simulink subsystem "Plant_Model_LTHT_Cooling"  (R2023a)
settings: Solver=VariableStepAuto  StartTime=0.0  StopTime=10.0  RelTol=1e-3
values from neighbouring files (symbols this model uses):
  air_cp = 1004    [All_Properties.mat]    (also in cathode_subsystem_parameters.m; thermal_subsystem_parameters.m)
  air_HC_min = 10    [All_Properties.mat]    (also in cathode_subsystem_parameters.m; thermal_subsystem_parameters.m)
  air_HC_nom = 100    [All_Properties.mat]    (also in cathode_subsystem_parameters.m; thermal_subsystem_parameters.m)
  air_rho = 1.2    [All_Properties.mat]    (also in cathode_subsystem_parameters.m; thermal_subsystem_parameters.m)
  air_vel_nom = 1    [All_Properties.mat]    (also in cathode_subsystem_parameters.m; thermal_subsystem_parameters.m)
  coolant_initial_pressure = 0.111325    [All_Properties.mat]    (also in cathode_subsystem_parameters.m; thermal_subsystem_parameters.m)
  coolant_initial_temperature = 313.15    [All_Properties.mat]    (also in cathode_subsystem_parameters.m = 293.15; thermal_subsystem_parameters.m = 293.15)
  coolant_tube_D = 0.05    [All_Properties.mat]    (also in Plant_Model_HT_Cooling_Parameters.m; cathode_subsystem_parameters.m; environment_parameters.m; stack_model_harness_parameters.m)
  radiator_area_air = 0.1026    [All_Properties.mat]    (also in cathode_subsystem_parameters.m; thermal_subsystem_parameters.m)
  radiator_area_fins = 2.543625    [All_Properties.mat]    (also in cathode_subsystem_parameters.m; thermal_subsystem_parameters.m)
  radiator_area_primary = 0.444525    [All_Properties.mat]    (also in cathode_subsystem_parameters.m; thermal_subsystem_parameters.m = 2 * radiator_tube_length * radiator_width * (radiator_fin_ro)
  radiator_n_tubes = 20    [All_Properties.mat]    (also in cathode_subsystem_parameters.m; thermal_subsystem_parameters.m)
  radiator_tube_height = 0.0015    [All_Properties.mat]    (also in cathode_subsystem_parameters.m; thermal_subsystem_parameters.m)
  radiator_tube_length = 0.45    [All_Properties.mat]    (also in cathode_subsystem_parameters.m; thermal_subsystem_parameters.m)
  radiator_width = 0.025    [All_Properties.mat]    (also in cathode_subsystem_parameters.m; thermal_subsystem_parameters.m)
  tcp_time_constant = 2    [All_Properties.mat]    (also in Plant_Model_HT_Cooling_Parameters.m; cathode_subsystem_parameters.m; thermal_subsystem_parameters.m)
  tcv_orifice_diameter = 0.045    [All_Properties.mat]    (also in Plant_Model_HT_Cooling_Parameters.m; cathode_subsystem_parameters.m; thermal_subsystem_parameters.m)
  tcv_time_constant = 0.2    [All_Properties.mat]    (also in Plant_Model_HT_Cooling_Parameters.m; cathode_subsystem_parameters.m; thermal_subsystem_parameters.m)
libraries: fl_lib x78, nesl_utility x61, SimscapeFluids_lib x9
(part 2 of 2)

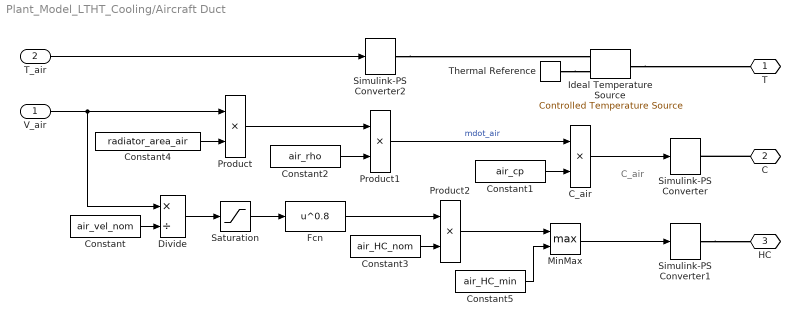
== system Plant_Model_LTHT_Cooling/Aircraft Duct ==
  note: C_air
  V_air : Inport
  T_air : Inport  Port=2
  C_air : Product
  Constant : Constant  Value=air_vel_nom
  Constant1 : Constant  Value=air_cp
  Constant2 : Constant  Value=air_rho
  Constant3 : Constant  Value=air_HC_nom
  Constant4 : Constant  Value=radiator_area_air
  Constant5 : Constant  Value=air_HC_min
  Divide : Product  Inputs=*/
  Fcn : Fcn  Expr=u^0.8
  Ideal Temperature Source : fl_lib/Thermal/Thermal Sources/Controlled Temperature Source
  MinMax : MinMax  Function=max  Inputs=2
  Product : Product
  Product1 : Product
  Product2 : Product
  Saturation : Saturate  UpperLimit=inf  LowerLimit=0
  Simulink-PS Converter : nesl_utility/Simulink-PS Converter  PhysicalDomain=network_engine_domain  SubClassName=ps_input  LeftPortType=input  RightPortType=output  PseudoPeriodic=off  Frequencies=[]  NoiseDistribution=none  NoiseParameters=[]  Unit=W/K  AffineConversion=off  FilteringAndDerivatives=zero  SimscapeFilterOrder=1  InputFilterTimeConstant=1  UdotUserProvided=1
  Simulink-PS Converter1 : nesl_utility/Simulink-PS Converter  PhysicalDomain=network_engine_domain  SubClassName=ps_input  LeftPortType=input  RightPortType=output  PseudoPeriodic=off  Frequencies=[]  NoiseDistribution=none  NoiseParameters=[]  Unit=W/(m^2*K)  AffineConversion=off  FilteringAndDerivatives=zero  SimscapeFilterOrder=1  InputFilterTimeConstant=1  UdotUserProvided=1
  Simulink-PS Converter2 : nesl_utility/Simulink-PS Converter  PhysicalDomain=network_engine_domain  SubClassName=ps_input  LeftPortType=input  RightPortType=output  PseudoPeriodic=off  Frequencies=[]  NoiseDistribution=none  NoiseParameters=[]  Unit=K  AffineConversion=on  FilteringAndDerivatives=zero  SimscapeFilterOrder=1  InputFilterTimeConstant=1  UdotUserProvided=1
  Thermal Reference : fl_lib/Thermal/Thermal Elements/Thermal Reference
  T : PMIOPort  Side=Right
  C : PMIOPort  Port=2  Side=Right
  HC : PMIOPort  Port=3  Side=Right
  wires:
  Saturation/1 -> Fcn/1
  Product1/1 -> C_air/1  "mdot_air"
  Constant4/1 -> Product/2
  Constant2/1 -> Product1/2
  Product/1 -> Product1/1
  C_air/1 -> Simulink-PS Converter/1
  Constant1/1 -> C_air/2
  T_air/1 -> Simulink-PS Converter2/1
  MinMax/1 -> Simulink-PS Converter1/1
  Constant5/1 -> MinMax/2
  Product2/1 -> MinMax/1
  Fcn/1 -> Product2/1
  Divide/1 -> Saturation/1
  Constant3/1 -> Product2/2
  Constant/1 -> Divide/2
  V_air/1 -> Divide/1, Product/1
  connections:
  Ideal Temperature Source/LConn1 -- T/RConn1
  Simulink-PS Converter2/RConn1 -- Ideal Temperature Source/RConn1
  Thermal Reference/LConn1 -- Ideal Temperature Source/RConn2
  Simulink-PS Converter1/RConn1 -- HC/RConn1
  C/RConn1 -- Simulink-PS Converter/RConn1

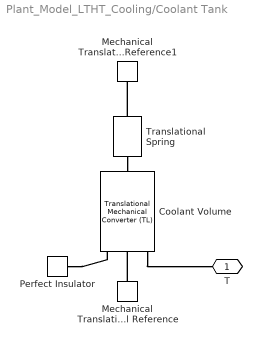
== system Plant_Model_LTHT_Cooling/Coolant Tank ==
  Coolant Volume : fl_lib/Thermal Liquid/Elements/Translational Mechanical Converter (TL)  mech_orientation=foundation.enum.MechOrientationTranslational.Positive  displacement_spec=foundation.enum.DisplacementSpec.Calculate  x0=x_init m  interface_area=A m^2  dead_volume=A * 0.001 m^3  environment_spec=foundation.enum.pressure_spec.specified  environment_pressure=coolant_initial_pressure MPa  dynamic_compressibility=simscape.enum.onoff.off  p0=env_p MPa  T0=coolant_initial_temperature K
      settings: InternalSimscapePortConfiguration="{\"Bottom\":[],\"Left\":[{\"id\":\"A\",\"label\":\"A\",\"type\":\"foundation.thermal_liquid.thermal_liquid\"},{\"id\":\"C\",\"label\":\"C\",\"type\":\"foundation.mechanical.translational.translational\"},{\"id\":\"H\",\"label\":\"H\",\"type\":\"foundation.thermal.thermal\"}],\"Right\":[{\"id\":\"R\",\"label\":\"R\",\"type\":\"foundation.mechanical.translational.translational\"}],\"Top\":[]}"
  Mechanical Translational Reference : fl_lib/Mechanical/Translational Elements/Mechanical Translational Reference
  Mechanical Translational Reference1 : fl_lib/Mechanical/Translational Elements/Mechanical Translational Reference
  Perfect Insulator : fl_lib/Thermal/Thermal Elements/Perfect Insulator  T_specify=off  T_priority=None  T=0 K  T_nominal_specify=off  T_nominal_unit=K  T_nominal_value=1
  Translational Spring : fl_lib/Mechanical/Translational Elements/Translational Spring  spr_rate=1e6 N/m  v_specify=off  v_priority=None  v=0 m/s  v_nominal_specify=off  v_nominal_unit=m/s  v_nominal_value=1  f_specify=off  f_priority=None  f=0 N  f_nominal_specify=off  f_nominal_unit=N  f_nominal_value=1  x_specify=off  x_priority=High  x=x_init m  x_nominal_specify=on  x_nominal_unit=m  x_nominal_value=x_init
  T : PMIOPort  Side=Right
  connections:
  Translational Spring/LConn1 -- Mechanical Translational Reference1/LConn1
  Translational Spring/RConn1 -- Coolant Volume/RConn1
  Perfect Insulator/LConn1 -- Coolant Volume/LConn3
  Mechanical Translational Reference/LConn1 -- Coolant Volume/LConn2
  Coolant Volume/LConn1 -- T/RConn1

== system Plant_Model_LTHT_Cooling/Kelvin to °C ==
  Temp. (K) : Inport
  Constant : Constant  Value=273.15
  Sum : Sum  Inputs=|+-
  Temp. (°C) : Outport
  wires:
  Temp. (K)/1 -> Sum/1
  Sum/1 -> Temp. (°C)/1
  Constant/1 -> Sum/2

== system Plant_Model_LTHT_Cooling/Kelvin to °C1 ==
  Temp. (K) : Inport
  Constant : Constant  Value=273.15
  Sum : Sum  Inputs=|+-
  Temp. (°C) : Outport
  wires:
  Temp. (K)/1 -> Sum/1
  Sum/1 -> Temp. (°C)/1
  Constant/1 -> Sum/2

== system Plant_Model_LTHT_Cooling/Kelvin to °C2 ==
  Temp. (K) : Inport
  Constant : Constant  Value=273.15
  Sum : Sum  Inputs=|+-
  Temp. (°C) : Outport
  wires:
  Temp. (K)/1 -> Sum/1
  Sum/1 -> Temp. (°C)/1
  Constant/1 -> Sum/2

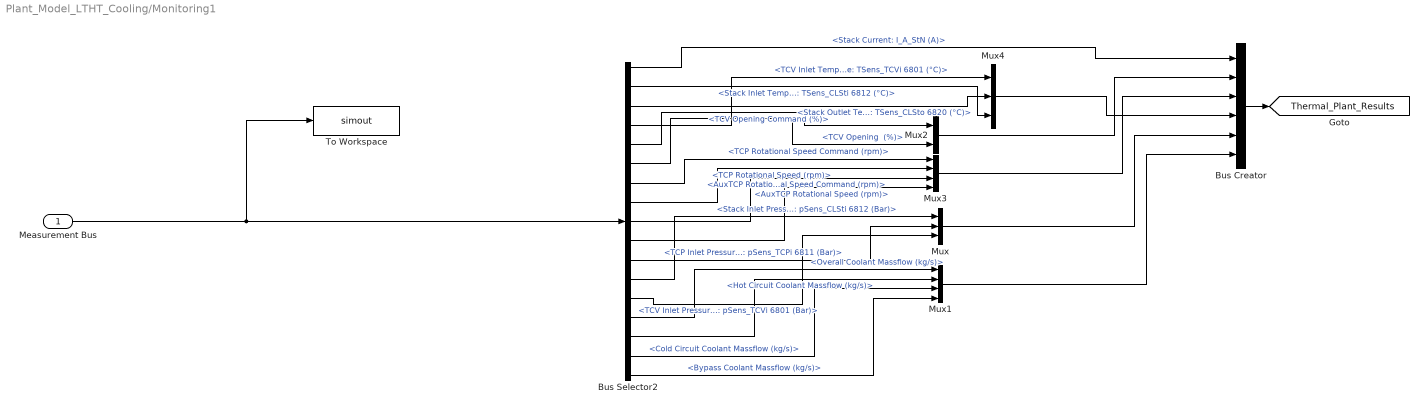
== system Plant_Model_LTHT_Cooling/Monitoring1 ==
  Measurement Bus : Inport
  Bus Creator : BusCreator  Inputs=6
  Bus Selector2 : BusSelector  OutputSignals="Stack Current: I_A_StN (A),Stack Inlet Temperature: TSens_CLSti 6812 (°C),Stack Outlet Temperature: TSens_CLSto 6820 (°C),TCV Inlet Temperature: TSens_TCVi 6801 (°C),TCV Opening Command (%),TCV Opening  (%),TCP Rotational Speed Command (rpm),TCP Rotational Speed (rpm),AuxTCP Rotational Speed Command (rpm),AuxTCP Rotational Speed (rpm),TCP Inlet Pressure: pSens_TCPi 6811 (Bar),Stack Inlet Pressure: pSens_CLSti 6812 (Bar),TCV Inlet Pressure: pSens_TCVi 6801 (Bar),Overall Coolant Massflow (kg/s),Hot Circuit Coolant Massflow (kg/s),Cold Circuit Coolant Massflow (kg/s),Bypass Coolant Massflow (kg/s)"
  Mux : Mux  Inputs=3
  Mux1 : Mux
  Mux2 : Mux  Inputs=2
  Mux3 : Mux
  Mux4 : Mux  Inputs=3
  To Workspace : ToWorkspace  VariableName=simout  SaveFormat=Timeseries  SampleTime=-1
  tag scope: Thermal_Plant_Results=global
  wires:
  Bus Creator/1 -> [Thermal_Plant_Results]
  Bus Selector2/4 -> Mux4/1  "<TCV Inlet Temperature: TSens_TCVi 6801 (°C)>"
  Bus Selector2/1 -> Bus Creator/1  "<Stack Current: I_A_StN (A)>"
  Bus Selector2/12 -> Mux/1  "<Stack Inlet Pressure: pSens_CLSti 6812 (Bar)>"
  Bus Selector2/16 -> Mux1/3  "<Cold Circuit Coolant Massflow (kg/s)>"
  Bus Selector2/5 -> Mux2/1  "<TCV Opening Command (%)>"
  Bus Selector2/8 -> Mux3/2  "<TCP Rotational Speed (rpm)>"
  Bus Selector2/17 -> Mux1/4  "<Bypass Coolant Massflow (kg/s)>"
  Mux1/1 -> Bus Creator/6
  Bus Selector2/14 -> Mux1/1  "<Overall Coolant Massflow (kg/s)>"
  Bus Selector2/13 -> Mux/3  "<TCV Inlet Pressure: pSens_TCVi 6801 (Bar)>"
  Bus Selector2/15 -> Mux1/2  "<Hot Circuit Coolant Massflow (kg/s)>"
  Mux/1 -> Bus Creator/5
  Bus Selector2/6 -> Mux2/2  "<TCV Opening  (%)>"
  Bus Selector2/2 -> Mux4/3  "<Stack Inlet Temperature: TSens_CLSti 6812 (°C)>"
  Bus Selector2/9 -> Mux3/3  "<AuxTCP Rotational Speed Command (rpm)>"
  Measurement Bus/1 -> Bus Selector2/1, To Workspace/1
  Mux2/1 -> Bus Creator/2
  Bus Selector2/3 -> Mux4/2  "<Stack Outlet Temperature: TSens_CLSto 6820 (°C)>"
  Bus Selector2/7 -> Mux3/1  "<TCP Rotational Speed Command (rpm)>"
  Mux3/1 -> Bus Creator/3
  Bus Selector2/11 -> Mux/2  "<TCP Inlet Pressure: pSens_TCPi 6811 (Bar)>"
  Mux4/1 -> Bus Creator/4
  Bus Selector2/10 -> Mux3/4  "<AuxTCP Rotational Speed (rpm)>"

== system Plant_Model_LTHT_Cooling/Pascal to Bar(a) ==
  Press. (Pa) : Inport
  Pa to Bar(a) : Gain  Gain=1e-5
  Press. Bar(a) : Outport
  wires:
  Press. (Pa)/1 -> Pa to Bar(a)/1
  Pa to Bar(a)/1 -> Press. Bar(a)/1

== system Plant_Model_LTHT_Cooling/Pascal to Bar(a)1 ==
  Press. (Pa) : Inport
  Pa to Bar(a) : Gain  Gain=1e-5
  Press. Bar(a) : Outport
  wires:
  Press. (Pa)/1 -> Pa to Bar(a)/1
  Pa to Bar(a)/1 -> Press. Bar(a)/1

== system Plant_Model_LTHT_Cooling/Pascal to Bar(a)2 ==
  Press. (Pa) : Inport
  Pa to Bar(a) : Gain  Gain=1e-5
  Press. Bar(a) : Outport
  wires:
  Press. (Pa)/1 -> Pa to Bar(a)/1
  Pa to Bar(a)/1 -> Press. Bar(a)/1

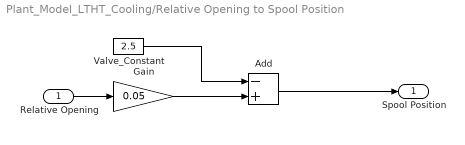
== system Plant_Model_LTHT_Cooling/Relative Opening to Spool Position ==
  Relative Opening : Inport
  Add : Sum  Inputs=-+
  Gain : Gain  Gain=0.05
  Valve_Constant : Constant  Value=2.5
  Spool Position : Outport
  wires:
  Add/1 -> Spool Position/1
  Valve_Constant/1 -> Add/1
  Relative Opening/1 -> Gain/1
  Gain/1 -> Add/2

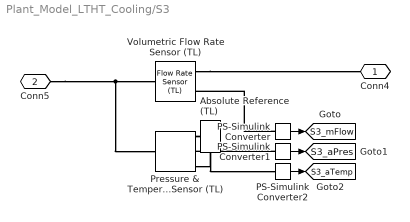
== system Plant_Model_LTHT_Cooling/S3 ==
  Absolute Reference (TL) : fl_lib/Thermal Liquid/Elements/Absolute Reference (TL)
  PS-Simulink Converter : nesl_utility/PS-Simulink Converter  PhysicalDomain=network_engine_domain  SubClassName=ps_output  LeftPortType=input  RightPortType=output  PseudoPeriodic=off  Frequencies=[]  VectorFormat=inherit  Unit=inherit  AffineConversion=off
  PS-Simulink Converter1 : nesl_utility/PS-Simulink Converter  PhysicalDomain=network_engine_domain  SubClassName=ps_output  LeftPortType=input  RightPortType=output  PseudoPeriodic=off  Frequencies=[]  VectorFormat=inherit  Unit=inherit  AffineConversion=off
  PS-Simulink Converter2 : nesl_utility/PS-Simulink Converter  PhysicalDomain=network_engine_domain  SubClassName=ps_output  LeftPortType=input  RightPortType=output  PseudoPeriodic=off  Frequencies=[]  VectorFormat=inherit  Unit=inherit  AffineConversion=off
  Pressure & Temperature Sensor (TL) : fl_lib/Thermal Liquid/Sensors/Pressure & Temperature Sensor (TL)  reference=foundation.enum.MeasurementReference.difference  pressure=true  pressure_spec=foundation.enum.PressureMeasementSpec.Absolute  temperature=true
      settings: LogSimulationData=on  InternalSimscapePortConfiguration="{\"Bottom\":[{\"id\":\"T\",\"label\":\"T\",\"type\":\"output\"}],\"Left\":[{\"id\":\"A\",\"label\":\"A\",\"type\":\"foundation.thermal_liquid.thermal_liquid\"}],\"Right\":[{\"id\":\"B\",\"label\":\"B\",\"type\":\"foundation.thermal_liquid.thermal_liquid\"},{\"id\":\"P\",\"label\":\"P\",\"type\":\"output\"}],\"Top\":[]}"
  Volumetric Flow Rate Sensor (TL) : fl_lib/Thermal Liquid/Sensors/Flow Rate Sensor (TL)  mass_flow_measure=false  volumetric_flow_measure=true  energy_flow_measure=false
      settings: InternalSimscapePortConfiguration="{\"Bottom\":[],\"Left\":[{\"id\":\"A\",\"label\":\"A\",\"type\":\"foundation.thermal_liquid.thermal_liquid\"}],\"Right\":[{\"id\":\"B\",\"label\":\"B\",\"type\":\"foundation.thermal_liquid.thermal_liquid\"},{\"id\":\"V\",\"label\":\"V\",\"type\":\"output\"}],\"Top\":[]}"
  Conn4 : PMIOPort  Side=Left
  Conn5 : PMIOPort  Port=2  Side=Right
  tag scope: S3_aPres=global, S3_aTemp=global, S3_mFlow=global
  wires:
  PS-Simulink Converter/1 -> [S3_mFlow]
  PS-Simulink Converter2/1 -> [S3_aTemp]
  PS-Simulink Converter1/1 -> [S3_aPres]
  connections:
  Conn5/RConn1 -- Pressure & Temperature Sensor (TL)/LConn1 -- Volumetric Flow Rate Sensor (TL)/LConn1
  Pressure & Temperature Sensor (TL)/RConn3 -- PS-Simulink Converter2/LConn1
  PS-Simulink Converter1/LConn1 -- Pressure & Temperature Sensor (TL)/RConn2
  Volumetric Flow Rate Sensor (TL)/RConn1 -- Conn4/RConn1
  PS-Simulink Converter/LConn1 -- Volumetric Flow Rate Sensor (TL)/RConn2
  Absolute Reference (TL)/LConn1 -- Pressure & Temperature Sensor (TL)/RConn1

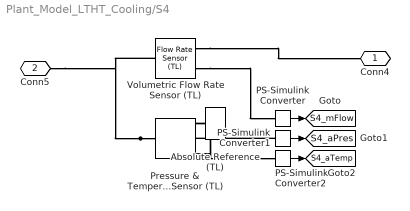
== system Plant_Model_LTHT_Cooling/S4 ==
  Absolute Reference (TL) : fl_lib/Thermal Liquid/Elements/Absolute Reference (TL)
  PS-Simulink Converter : nesl_utility/PS-Simulink Converter  PhysicalDomain=network_engine_domain  SubClassName=ps_output  LeftPortType=input  RightPortType=output  PseudoPeriodic=off  Frequencies=[]  VectorFormat=inherit  Unit=inherit  AffineConversion=off
  PS-Simulink Converter1 : nesl_utility/PS-Simulink Converter  PhysicalDomain=network_engine_domain  SubClassName=ps_output  LeftPortType=input  RightPortType=output  PseudoPeriodic=off  Frequencies=[]  VectorFormat=inherit  Unit=inherit  AffineConversion=off
  PS-Simulink Converter2 : nesl_utility/PS-Simulink Converter  PhysicalDomain=network_engine_domain  SubClassName=ps_output  LeftPortType=input  RightPortType=output  PseudoPeriodic=off  Frequencies=[]  VectorFormat=inherit  Unit=inherit  AffineConversion=off
  Pressure & Temperature Sensor (TL) : fl_lib/Thermal Liquid/Sensors/Pressure & Temperature Sensor (TL)  reference=foundation.enum.MeasurementReference.difference  pressure=true  pressure_spec=foundation.enum.PressureMeasementSpec.Absolute  temperature=true
      settings: InternalSimscapePortConfiguration="{\"Bottom\":[{\"id\":\"T\",\"label\":\"T\",\"type\":\"output\"}],\"Left\":[{\"id\":\"A\",\"label\":\"A\",\"type\":\"foundation.thermal_liquid.thermal_liquid\"}],\"Right\":[{\"id\":\"B\",\"label\":\"B\",\"type\":\"foundation.thermal_liquid.thermal_liquid\"},{\"id\":\"P\",\"label\":\"P\",\"type\":\"output\"}],\"Top\":[]}"
  Volumetric Flow Rate Sensor (TL) : fl_lib/Thermal Liquid/Sensors/Flow Rate Sensor (TL)  mass_flow_measure=false  volumetric_flow_measure=true  energy_flow_measure=false
      settings: InternalSimscapePortConfiguration="{\"Bottom\":[],\"Left\":[{\"id\":\"A\",\"label\":\"A\",\"type\":\"foundation.thermal_liquid.thermal_liquid\"}],\"Right\":[{\"id\":\"B\",\"label\":\"B\",\"type\":\"foundation.thermal_liquid.thermal_liquid\"},{\"id\":\"V\",\"label\":\"V\",\"type\":\"output\"}],\"Top\":[]}"
  Conn4 : PMIOPort  Side=Left
  Conn5 : PMIOPort  Port=2  Side=Right
  tag scope: S4_aPres=global, S4_aTemp=global, S4_mFlow=global
  wires:
  PS-Simulink Converter1/1 -> [S4_aPres]
  PS-Simulink Converter2/1 -> [S4_aTemp]
  PS-Simulink Converter/1 -> [S4_mFlow]
  connections:
  Volumetric Flow Rate Sensor (TL)/RConn2 -- PS-Simulink Converter/LConn1
  Volumetric Flow Rate Sensor (TL)/RConn1 -- Conn4/RConn1
  PS-Simulink Converter1/LConn1 -- Pressure & Temperature Sensor (TL)/RConn2
  Pressure & Temperature Sensor (TL)/RConn3 -- PS-Simulink Converter2/LConn1
  Pressure & Temperature Sensor (TL)/LConn1 -- Volumetric Flow Rate Sensor (TL)/LConn1 -- Conn5/RConn1
  Absolute Reference (TL)/LConn1 -- Pressure & Temperature Sensor (TL)/RConn1

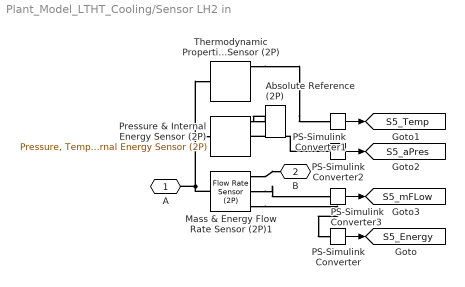
== system Plant_Model_LTHT_Cooling/Sensor LH2 in ==
  Absolute Reference (2P) : fl_lib/Two-Phase Fluid/Elements/Absolute Reference (2P)
  Mass & Energy Flow Rate Sensor (2P)1 : fl_lib/Two-Phase Fluid/Sensors/Flow Rate Sensor (2P)  mass_flow_measure=true  volumetric_flow_measure=false  energy_flow_measure=true
      settings: InternalSimscapePortConfiguration="{\"Bottom\":[{\"id\":\"PHI\",\"label\":\"φ\",\"type\":\"output\"}],\"Left\":[{\"id\":\"A\",\"label\":\"A\",\"type\":\"foundation.two_phase_fluid.two_phase_fluid\"}],\"Right\":[{\"id\":\"B\",\"label\":\"B\",\"type\":\"foundation.two_phase_fluid.two_phase_fluid\"},{\"id\":\"M\",\"label\":\"M\",\"type\":\"output\"}],\"Top\":[]}"
  PS-Simulink Converter : nesl_utility/PS-Simulink Converter  PhysicalDomain=network_engine_domain  SubClassName=ps_output  LeftPortType=input  RightPortType=output  PseudoPeriodic=off  Frequencies=[]  VectorFormat=inherit  Unit=kW  AffineConversion=off
  PS-Simulink Converter1 : nesl_utility/PS-Simulink Converter  PhysicalDomain=network_engine_domain  SubClassName=ps_output  LeftPortType=input  RightPortType=output  PseudoPeriodic=off  Frequencies=[]  VectorFormat=1-D array  Unit=inherit  AffineConversion=off
  PS-Simulink Converter2 : nesl_utility/PS-Simulink Converter  PhysicalDomain=network_engine_domain  SubClassName=ps_output  LeftPortType=input  RightPortType=output  PseudoPeriodic=off  Frequencies=[]  VectorFormat=1-D array  Unit=inherit  AffineConversion=off
  PS-Simulink Converter3 : nesl_utility/PS-Simulink Converter  PhysicalDomain=network_engine_domain  SubClassName=ps_output  LeftPortType=input  RightPortType=output  PseudoPeriodic=off  Frequencies=[]  VectorFormat=1-D array  Unit=inherit  AffineConversion=off
  Pressure & Internal Energy Sensor (2P) : fl_lib/Two-Phase Fluid/Sensors/Pressure, Temperature & Internal Energy Sensor (2P)  reference=foundation.enum.MeasurementReference.difference  pressure=true  pressure_spec=foundation.enum.PressureMeasementSpec.Absolute  temperature=false  internal_energy=true
      settings: InternalSimscapePortConfiguration="{\"Bottom\":[{\"id\":\"U\",\"label\":\"U\",\"type\":\"output\"}],\"Left\":[{\"id\":\"A\",\"label\":\"A\",\"type\":\"foundation.two_phase_fluid.two_phase_fluid\"}],\"Right\":[{\"id\":\"B\",\"label\":\"B\",\"type\":\"foundation.two_phase_fluid.two_phase_fluid\"},{\"id\":\"P\",\"label\":\"P\",\"type\":\"output\"}],\"Top\":[]}"
  Thermodynamic Properties Sensor (2P) : fl_lib/Two-Phase Fluid/Sensors/Thermodynamic Properties Sensor (2P)  temperature=true  enthalpy=true  density=false  specific_volume=true  entropy=true
      settings: InternalSimscapePortConfiguration="{\"Bottom\":[{\"id\":\"V\",\"label\":\"v\",\"type\":\"output\"},{\"id\":\"S\",\"label\":\"s\",\"type\":\"output\"}],\"Left\":[{\"id\":\"A\",\"label\":\"A\",\"type\":\"foundation.two_phase_fluid.two_phase_fluid\"}],\"Right\":[{\"id\":\"T\",\"label\":\"T\",\"type\":\"output\"},{\"id\":\"H\",\"label\":\"h\",\"type\":\"output\"}],\"Top\":[]}"
  A : PMIOPort  Side=Left
  B : PMIOPort  Port=2  Side=Right
  tag scope: S5_Energy=global, S5_Temp=global, S5_aPres=global, S5_mFLow=global
  wires:
  PS-Simulink Converter/1 -> [S5_Energy]
  PS-Simulink Converter1/1 -> [S5_Temp]
  PS-Simulink Converter2/1 -> [S5_aPres]
  PS-Simulink Converter3/1 -> [S5_mFLow]
  connections:
  Mass & Energy Flow Rate Sensor (2P)1/RConn1 -- B/RConn1
  A/RConn1 -- Thermodynamic Properties Sensor (2P)/LConn1 -- Pressure & Internal Energy Sensor (2P)/LConn1 -- Mass & Energy Flow Rate Sensor (2P)1/LConn1
  Mass & Energy Flow Rate Sensor (2P)1/RConn3 -- PS-Simulink Converter/LConn1
  Thermodynamic Properties Sensor (2P)/RConn1 -- PS-Simulink Converter1/LConn1
  PS-Simulink Converter2/LConn1 -- Pressure & Internal Energy Sensor (2P)/RConn2
  Mass & Energy Flow Rate Sensor (2P)1/RConn2 -- PS-Simulink Converter3/LConn1
  Pressure & Internal Energy Sensor (2P)/RConn1 -- Absolute Reference (2P)/LConn1

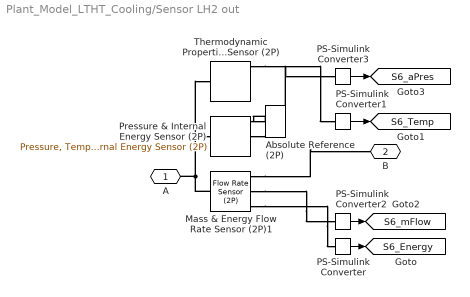
== system Plant_Model_LTHT_Cooling/Sensor LH2 out ==
  Absolute Reference (2P) : fl_lib/Two-Phase Fluid/Elements/Absolute Reference (2P)
  Mass & Energy Flow Rate Sensor (2P)1 : fl_lib/Two-Phase Fluid/Sensors/Flow Rate Sensor (2P)  mass_flow_measure=true  volumetric_flow_measure=false  energy_flow_measure=true
      settings: InternalSimscapePortConfiguration="{\"Bottom\":[{\"id\":\"PHI\",\"label\":\"φ\",\"type\":\"output\"}],\"Left\":[{\"id\":\"A\",\"label\":\"A\",\"type\":\"foundation.two_phase_fluid.two_phase_fluid\"}],\"Right\":[{\"id\":\"B\",\"label\":\"B\",\"type\":\"foundation.two_phase_fluid.two_phase_fluid\"},{\"id\":\"M\",\"label\":\"M\",\"type\":\"output\"}],\"Top\":[]}"
  PS-Simulink Converter : nesl_utility/PS-Simulink Converter  PhysicalDomain=network_engine_domain  SubClassName=ps_output  LeftPortType=input  RightPortType=output  PseudoPeriodic=off  Frequencies=[]  VectorFormat=1-D array  Unit=kW  AffineConversion=off
  PS-Simulink Converter1 : nesl_utility/PS-Simulink Converter  PhysicalDomain=network_engine_domain  SubClassName=ps_output  LeftPortType=input  RightPortType=output  PseudoPeriodic=off  Frequencies=[]  VectorFormat=1-D array  Unit=degC  AffineConversion=off
  PS-Simulink Converter2 : nesl_utility/PS-Simulink Converter  PhysicalDomain=network_engine_domain  SubClassName=ps_output  LeftPortType=input  RightPortType=output  PseudoPeriodic=off  Frequencies=[]  VectorFormat=1-D array  Unit=1  AffineConversion=off
  PS-Simulink Converter3 : nesl_utility/PS-Simulink Converter  PhysicalDomain=network_engine_domain  SubClassName=ps_output  LeftPortType=input  RightPortType=output  PseudoPeriodic=off  Frequencies=[]  VectorFormat=1-D array  Unit=inherit  AffineConversion=off
  Pressure & Internal Energy Sensor (2P) : fl_lib/Two-Phase Fluid/Sensors/Pressure, Temperature & Internal Energy Sensor (2P)  reference=foundation.enum.MeasurementReference.difference  pressure=true  pressure_spec=foundation.enum.PressureMeasementSpec.Absolute  temperature=false  internal_energy=true
      settings: InternalSimscapePortConfiguration="{\"Bottom\":[{\"id\":\"U\",\"label\":\"U\",\"type\":\"output\"}],\"Left\":[{\"id\":\"A\",\"label\":\"A\",\"type\":\"foundation.two_phase_fluid.two_phase_fluid\"}],\"Right\":[{\"id\":\"B\",\"label\":\"B\",\"type\":\"foundation.two_phase_fluid.two_phase_fluid\"},{\"id\":\"P\",\"label\":\"P\",\"type\":\"output\"}],\"Top\":[]}"
  Thermodynamic Properties Sensor (2P) : fl_lib/Two-Phase Fluid/Sensors/Thermodynamic Properties Sensor (2P)  temperature=true  enthalpy=true  density=false  specific_volume=true  entropy=true
      settings: InternalSimscapePortConfiguration="{\"Bottom\":[{\"id\":\"V\",\"label\":\"v\",\"type\":\"output\"},{\"id\":\"S\",\"label\":\"s\",\"type\":\"output\"}],\"Left\":[{\"id\":\"A\",\"label\":\"A\",\"type\":\"foundation.two_phase_fluid.two_phase_fluid\"}],\"Right\":[{\"id\":\"T\",\"label\":\"T\",\"type\":\"output\"},{\"id\":\"H\",\"label\":\"h\",\"type\":\"output\"}],\"Top\":[]}"
  A : PMIOPort  Side=Left
  B : PMIOPort  Port=2  Side=Right
  tag scope: S6_Energy=global, S6_Temp=global, S6_aPres=global, S6_mFlow=global
  wires:
  PS-Simulink Converter1/1 -> [S6_Temp]
  PS-Simulink Converter/1 -> [S6_Energy]
  PS-Simulink Converter2/1 -> [S6_mFlow]
  PS-Simulink Converter3/1 -> [S6_aPres]
  connections:
  Mass & Energy Flow Rate Sensor (2P)1/RConn3 -- PS-Simulink Converter/LConn1
  Mass & Energy Flow Rate Sensor (2P)1/RConn1 -- B/RConn1
  Thermodynamic Properties Sensor (2P)/RConn1 -- PS-Simulink Converter1/LConn1
  Mass & Energy Flow Rate Sensor (2P)1/RConn2 -- PS-Simulink Converter2/LConn1
  Pressure & Internal Energy Sensor (2P)/RConn2 -- PS-Simulink Converter3/LConn1
  A/RConn1 -- Thermodynamic Properties Sensor (2P)/LConn1 -- Pressure & Internal Energy Sensor (2P)/LConn1 -- Mass & Energy Flow Rate Sensor (2P)1/LConn1
  Pressure & Internal Energy Sensor (2P)/RConn1 -- Absolute Reference (2P)/LConn1

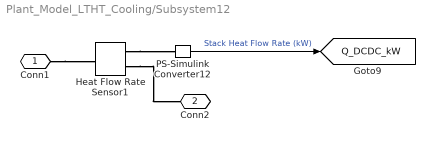
== system Plant_Model_LTHT_Cooling/Subsystem12 ==
  Heat Flow Rate Sensor1 : fl_lib/Thermal/Thermal Sensors/Heat Flow Rate Sensor
  PS-Simulink Converter12 : nesl_utility/PS-Simulink Converter  PhysicalDomain=network_engine_domain  SubClassName=ps_output  LeftPortType=input  RightPortType=output  PseudoPeriodic=off  Frequencies=[]  VectorFormat=1-D array  Unit=kW  AffineConversion=off
  Conn1 : PMIOPort  Side=Left
  Conn2 : PMIOPort  Port=2  Side=Right
  tag scope: Q_DCDC_kW=global
  wires:
  PS-Simulink Converter12/1 -> [Q_DCDC_kW]  "Stack Heat Flow Rate (kW)"
  connections:
  Heat Flow Rate Sensor1/RConn2 -- Conn2/RConn1
  Conn1/RConn1 -- Heat Flow Rate Sensor1/LConn1
  Heat Flow Rate Sensor1/RConn1 -- PS-Simulink Converter12/LConn1

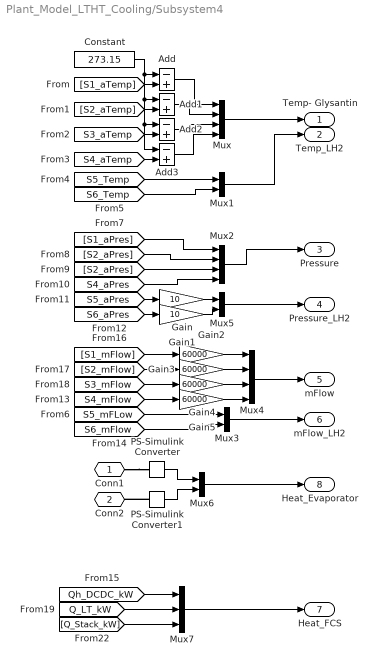
== system Plant_Model_LTHT_Cooling/Subsystem4 ==
  Add{,1..3} (4 alike) : Sum  Inputs=-+
  Constant : Constant  Value=273.15
  Gain : Gain  Gain=10
  Gain1 : Gain  Gain=10
  Gain{2..5} (4 alike) : Gain  Gain=60000
  Mux : Mux
  Mux{1,3,5..6} (4 alike) : Mux  Inputs=2
  Mux2 : Mux
  Mux4 : Mux
  Mux7 : Mux  Inputs=3
  PS-Simulink Converter : nesl_utility/PS-Simulink Converter  PhysicalDomain=network_engine_domain  SubClassName=ps_output  LeftPortType=input  RightPortType=output  PseudoPeriodic=off  Frequencies=[]  VectorFormat=inherit  Unit=inherit  AffineConversion=off
  PS-Simulink Converter1 : nesl_utility/PS-Simulink Converter  PhysicalDomain=network_engine_domain  SubClassName=ps_output  LeftPortType=input  RightPortType=output  PseudoPeriodic=off  Frequencies=[]  VectorFormat=inherit  Unit=inherit  AffineConversion=off
  Conn1 : PMIOPort  Side=Left
  Conn2 : PMIOPort  Port=2  Side=Left
  Temp- Glysantin : Outport
  Temp_LH2 : Outport  Port=2
  Pressure : Outport  Port=3
  Pressure_LH2 : Outport  Port=4
  mFlow : Outport  Port=5
  mFlow_LH2 : Outport  Port=6
  Heat_FCS : Outport  Port=7
  Heat_Evaporator : Outport  Port=8
  wires:
  [S4_aPres] -> Mux2/4
  [S2_mFlow] -> Gain3/1
  [S1_mFlow] -> Gain2/1
  [S2_aPres] -> Mux2/3
  [S3_mFlow] -> Gain4/1
  [S2_aPres] -> Mux2/2
  [S4_mFlow] -> Gain5/1
  [S1_aPres] -> Mux2/1
  [S6_mFlow] -> Mux3/2
  Mux4/1 -> mFlow/1
  Mux/1 -> Temp- Glysantin/1
  Mux1/1 -> Temp_LH2/1
  Mux2/1 -> Pressure/1
  [S1_aTemp] -> Add/2
  Constant/1 -> Add3/1, Add2/1, Add1/1, Add/1
  [S2_aTemp] -> Add1/2
  [S3_aTemp] -> Add2/2
  [S4_aTemp] -> Add3/2
  [S6_Temp] -> Mux1/2
  [S5_Temp] -> Mux1/1
  Add3/1 -> Mux/4
  Add2/1 -> Mux/3
  Add1/1 -> Mux/2
  Add/1 -> Mux/1
  [S5_mFLow] -> Mux3/1
  Mux3/1 -> mFlow_LH2/1
  [S6_aPres] -> Gain1/1
  Mux5/1 -> Pressure_LH2/1
  [S5_aPres] -> Gain/1
  Gain/1 -> Mux5/1
  Gain1/1 -> Mux5/2
  Gain2/1 -> Mux4/1
  Gain3/1 -> Mux4/2
  Gain4/1 -> Mux4/3
  Gain5/1 -> Mux4/4
  PS-Simulink Converter/1 -> Mux6/1
  PS-Simulink Converter1/1 -> Mux6/2
  Mux6/1 -> Heat_Evaporator/1
  [Qh_DCDC_kW] -> Mux7/1
  [Q_LT_kW] -> Mux7/2
  [Q_Stack_kW] -> Mux7/3
  Mux7/1 -> Heat_FCS/1
  connections:
  Conn1/RConn1 -- PS-Simulink Converter/LConn1
  PS-Simulink Converter1/LConn1 -- Conn2/RConn1

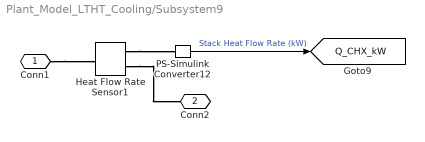
== system Plant_Model_LTHT_Cooling/Subsystem9 ==
  Heat Flow Rate Sensor1 : fl_lib/Thermal/Thermal Sensors/Heat Flow Rate Sensor
  PS-Simulink Converter12 : nesl_utility/PS-Simulink Converter  PhysicalDomain=network_engine_domain  SubClassName=ps_output  LeftPortType=input  RightPortType=output  PseudoPeriodic=off  Frequencies=[]  VectorFormat=1-D array  Unit=kW  AffineConversion=off
  Conn1 : PMIOPort  Side=Left
  Conn2 : PMIOPort  Port=2  Side=Right
  tag scope: Q_CHX_kW=global
  wires:
  PS-Simulink Converter12/1 -> [Q_CHX_kW]  "Stack Heat Flow Rate (kW)"
  connections:
  Heat Flow Rate Sensor1/RConn1 -- PS-Simulink Converter12/LConn1
  Conn1/RConn1 -- Heat Flow Rate Sensor1/LConn1
  Heat Flow Rate Sensor1/RConn2 -- Conn2/RConn1
